simulink model "week1problem5"  (R2020b)
settings: Solver=VariableStepAuto  StartTime=0.0  StopTime=10.0  RelTol=1e-3
model workspace (MAT data in the model file):
  C = 1e-05
  R = 10
settings Model: OrderedModelArguments=off  Creator=Puru Gawande  LastModifiedBy=Puru Gawande

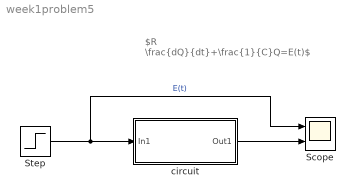
== system week1problem5 ==
  note: $R \frac{dQ}{dt}+\frac{1}{C}Q=E(t)$
  Scope : Scope  NumInputPorts=2
  Step : Step  Before=1  After=3  SampleTime=0
  circuit : Subsystem  TreatAsAtomicUnit=on
  wires:
  Step/1 -> Scope/1, circuit/1(In1)  "E(t)"
  circuit/1(Out1) -> Scope/2

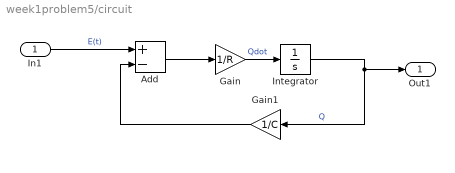
== system week1problem5/circuit ==
  In1 : Inport
  Add : Sum  Inputs=+-
  Gain : Gain  Gain=1/R
  Gain1 : Gain  Gain=1/C
  Integrator : Integrator  InitialCondition=8
  Out1 : Outport
  wires:
  In1/1 -> Add/1  "E(t)"
  Gain1/1 -> Add/2
  Gain/1 -> Integrator/1  "Qdot"
  Integrator/1 -> Out1/1, Gain1/1  "Q"
  Add/1 -> Gain/1
